simulink model "OQPSK"  (R2016a)
settings: Solver=VariableStepAuto  StartTime=0.0  StopTime=10.0  RelTol=1e-3
libraries: powerlib_meascontrol x1
settings Model: Creator=ASUS  LastModifiedBy=ASUS

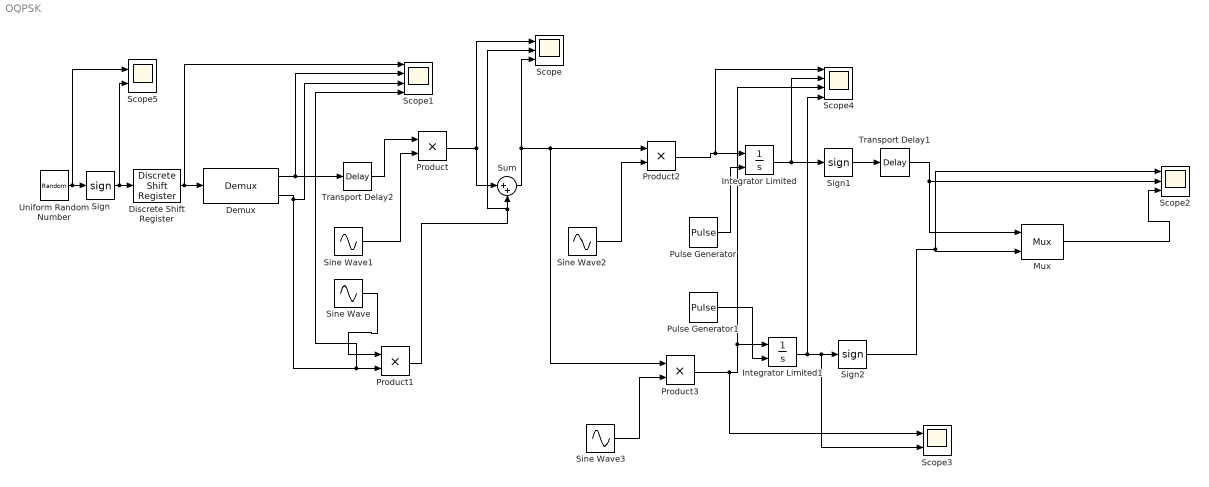
== system OQPSK ==
  Demux : Demux  Outputs=2
  Discrete Shift Register : powerlib_meascontrol/Additional Components/Discrete Shift Register  NSamples=2  InitialValue=0  Ts=1
  Integrator Limited : Integrator  ExternalReset=level  LimitOutput=on  UpperSaturationLimit=1  LowerSaturationLimit=0
  Integrator Limited1 : Integrator  ExternalReset=level  LimitOutput=on  UpperSaturationLimit=1  LowerSaturationLimit=0
  Mux : Mux  Inputs=2
  Product{,1..3} (4 alike) : Product
  Pulse Generator : DiscretePulseGenerator  PulseType=Time based  PhaseDelay=1  SampleTime=.01
  Pulse Generator1 : DiscretePulseGenerator  PulseType=Time based  PhaseDelay=1
  Scope : Scope  NumInputPorts=3
  Scope1 : Scope  NumInputPorts=4
  Scope2 : Scope  NumInputPorts=3
  Scope3 : Scope  NumInputPorts=2
  Scope4 : Scope  NumInputPorts=4
  Scope5 : Scope  NumInputPorts=2
  Sign : Signum
  Sign1 : Signum
  Sign2 : Signum
  Sine Wave : Sin  Frequency=2*pi*5  SampleTime=.01
  Sine Wave1 : Sin  Frequency=2*pi*5  Phase=pi/2  SampleTime=.01
  Sine Wave2 : Sin  Frequency=2*pi*5  Phase=pi/2  SampleTime=.01
  Sine Wave3 : Sin  Frequency=2*pi*5  SampleTime=.01
  Sum : Sum  Inputs=|++
  Transport Delay1 : TransportDelay
  Transport Delay2 : TransportDelay
  Uniform Random Number : UniformRandomNumber  SampleTime=1
  wires:
  Uniform Random Number/1 -> Scope5/1, Sign/1
  Sign/1 -> Scope5/2, Discrete Shift Register/1
  Discrete Shift Register/1 -> Scope1/1, Demux/1
  Product/1 -> Sum/1, Scope/1
  Product1/1 -> Scope/2, Sum/2
  Sine Wave1/1 -> Product/2
  Sine Wave/1 -> Product1/1
  Demux/1 -> Transport Delay2/1, Scope1/2
  Sum/1 -> Product3/1, Product2/1, Scope/3
  Sine Wave2/1 -> Product2/2
  Product2/1 -> Scope4/1, Integrator Limited/1
  Pulse Generator/1 -> Integrator Limited/2
  Product3/1 -> Integrator Limited1/1, Scope4/3, Scope3/1
  Integrator Limited1/1 -> Scope4/4, Scope3/2, Sign2/1
  Sign2/1 -> Mux/2, Scope2/1
  Integrator Limited/1 -> Sign1/1, Scope4/2
  Transport Delay1/1 -> Mux/1, Scope2/2
  Sine Wave3/1 -> Product3/2
  Pulse Generator1/1 -> Integrator Limited1/2
  Mux/1 -> Scope2/3
  Sign1/1 -> Transport Delay1/1
  Demux/2 -> Scope1/4, Product1/2, Scope1/3
  Transport Delay2/1 -> Product/1
